simulink model "EffectuatorIntegratedWithDemonstrator"  (R2020a)
settings: Solver=FixedStepDiscrete  StartTime=0.0  StopTime=inf  FixedStep=Ts  RelTol=1e-3
InitFcn:
  | %% Verwende vordefinierte Setpoints (Kreis mit Z-Komponente)
  | 
  | % Config
  | numCircles = 3;
  | scale=6;
  | %Versuch symmetrische Setpunkte zu setzen
  | pointsPerCircle =scale*(4+3*numCircles)+2;
  | 
  | r = 50;
  | m_x = r;
  | m_y = r;
  | 
  | % //
  | s = linspace(0,2*pi,pointsPerCircle);
  | 
  | setPoints_x = [];
  | setPoints_y = [];
  | 
  | for ii=1:numCircles
  | 
  | setPoints_x = [setPoints_x (-cos(s(1:floor(pointsPerCircle / 2))).*r + m_x + 2*r*(ii-1))]; %#ok<AGROW>
  | setPoints_y = [setPoints_y (sin(s).*r+m_y)]; %#ok<AGROW>pointsPerCircle / 2
  | 
  | end
  | 
  | setPoints_x = [setPoints_x flip(setPoints_x(1:end))];
  | 
  | % Loeschen doppelter y-Werte (Kreisuebergang)
  | setPoints_x(pointsPerCircle .* [1:numCircles]) = [];
  | setPoints_y(pointsPerCircle .* [1:numCircles]) = [];
  | 
  | % setPoints_x= [linspace(0,setPoints_x(19),19) setPoints_x(20:end)];
  | % setPoints_y= [linspace(0,setPoints_y(19),19) setPoints_y(20:end)];
  | 
  | % Array Elemente verschieben
  | % setPoints_x = circshift(setPoints_x,-pointsPerCircle/4,2);
  | % setPoints_y = circshift(setPoints_y,-pointsPerCircle/4,2);
  | 
  | z = zeros(1,size(setPoints_x,2));
  | z_x = -5:5;
  | z_y = -z_x.^2 + 25;
  | z_idx = 90;
  | z_idx2 = 210;
  | z(z_idx:z_idx+length(z_x)-1) = z_y;
  | z(z_idx2:z_idx2+length(z_x)-1) = z_y;
  | % z = [z_y z];
  | setPoints_z = z;
  | 
  | % setPoints_x = [zeros(1,length(z_y)) setPoints_x];
  | % setPoints_y = [setPoints_y(1,1)*ones(1,length(z_y)) setPoints_y];
  | 
  | % Umrechnung der Einheiten für Demonstrator
  | % setPoints_x = setPoints_x ./ 1000;
  | % setPoints_y = setPoints_y ./ 1000;
  | % setPoints_z = setPoints_z ./ 1000;
  | 
  | 
  | %{
  | plot(setPoints_x,setPoints_y);
  | fig = figure;
  | ... (+13 lines)
StartFcn:
  | close all;
model workspace (MAT data in the model file):
  MvmtPerfEval_collectVal : Simulink.Parameter (value not decoded)
  MvmtPerfEval_sendOwnVal : Simulink.Parameter (value not decoded)
  PerfEval_numTicks_enable : Simulink.Parameter (value not decoded)
  Segmentregler_I_Gain : Simulink.Parameter (value not decoded)
  Segmentregler_P_Gain : Simulink.Parameter (value not decoded)
  Segmentregler_minVel_enable : Simulink.Parameter (value not decoded)
  Segmentregler_numTicks_enable : Simulink.Parameter (value not decoded)
  Ts : Simulink.Parameter (value not decoded)
  maxPos_x : Simulink.Parameter (value not decoded)
  maxPos_y : Simulink.Parameter (value not decoded)
  maxPos_z : Simulink.Parameter (value not decoded)
  maxVectorLengths : Simulink.Parameter (value not decoded)
  minAllowedVelSaturation : Simulink.Parameter (value not decoded)
  numAxes : Simulink.Parameter (value not decoded)
symbols that are objects in the model workspace (value not decoded): maxPos_x, maxPos_y, maxPos_z, minAllowedVelSaturation, MvmtPerfEval_collectVal, MvmtPerfEval_sendOwnVal, numAxes, PerfEval_numTicks_enable, Segmentregler_I_Gain, Segmentregler_minVel_enable, Segmentregler_numTicks_enable, Segmentregler_P_Gain, Ts
undefined symbols (not defined in the file or in its folder): DiscIntNeverNeededParam, VelOverride
libraries: simulink x20, vrlib x5, sldrtlib x2, xpcrtudplib x2, dspnetwork x2, ptplib x1, etargetslib x1, xpcutilitieslib x1
(part 3 of 5)

== system EffectuatorIntegratedWithDemonstrator/Joystick Ctrl ==
  note: x-Achse
  note: y-Achse
  note: z-Achse
  Custom Gauge : CustomGaugeBlock  LabelPosition=Hide  NeedleImage=data:image/svg+xml;base64,PD94bWwgdmVyc2lvbj0iMS4wIiBlbmNvZGluZz0idXRmLTgiPz4KPCEtLSBHZW5lcmF0b3I6IEFkb2JlIElsbHVzdHJhdG9yIDE5LjIuMSwgU1ZHIEV4cG9ydCBQbHVnLUluIC4gU1ZHIFZlcnNpb246IDYuMDAgQnVpbGQgMCkgIC0tPgo8c3ZnIHZlcnNpb249IjEuMSIgeG1sbnM9Imh0dHA6Ly93d3cudzMub3JnLzIwMDAvc3ZnIiB4bWxuczp4bGluaz0iaHR0cDovL3d3dy53My5vcmcvMTk5OS94bGluayIgeD0iMHB4IiB5PSIwcHgiCgkgdmlld0JveD0iMCAwIDIwMCA1MCIgc3R5bGU9ImVuYWJsZS1iYWNrZ3JvdW5kOm5ldyAw ...(+9940 chars)  NeedleXPos=0.37269714818065863  NeedleYPos=0.4799889804603517  NeedleHeight=0.12331842798957203  NeedleWidth=0.20315800404452888  NeedleInitialRotation=-59.94322499147643  GaugeMax=1  GaugeArcDefined=true  GaugeArcRadius=0.14440076769366753  GaugeArcStrokeWidth=0.042228358658436646  GaugeArcRotation=240.5385250290321  GaugeArcRatio=0.8333333333333  GaugeArcTransparency=0  ValueArcTransparency=0  ValueArcColor=#1759b0  GaugeTickColor=#000000  ScaleColorsJSON=[]  IsLinearGauge=false  GaugeTrackLeft=0.35  GaugeTrackTop=0.35  GaugeTrackHeight=0.1  GaugeTrackWidth=0.3  GaugeTrackRotation=0
  Custom Gauge1 : CustomGaugeBlock  LabelPosition=Hide  GaugeMax=1  GaugeArcDefined=true  GaugeArcRadius=0.1358563990074277  GaugeArcStrokeWidth=0.03972965542329953  GaugeArcRotation=240.5385250290321  GaugeArcRatio=0.8333333333333  GaugeArcTransparency=0  ValueArcColor=#1759b0  GaugeTickColor=#000000  ScaleColorsJSON=[]  IsLinearGauge=false  GaugeTrackLeft=0.35  GaugeTrackTop=0.35  GaugeTrackHeight=0.1  GaugeTrackWidth=0.3  GaugeTrackRotation=0
  Custom Gauge2 : CustomGaugeBlock  LabelPosition=Hide  GaugeMax=1  GaugeArcDefined=true  GaugeArcRadius=0.1358563990074277  GaugeArcStrokeWidth=0.03972965542329953  GaugeArcRotation=240.5385250290321  GaugeArcRatio=0.8333333333333  GaugeArcTransparency=0  ValueArcColor=#1759b0  GaugeTickColor=#000000  ScaleColorsJSON=[]  IsLinearGauge=false  GaugeTrackLeft=0.35  GaugeTrackTop=0.35  GaugeTrackHeight=0.1  GaugeTrackWidth=0.3  GaugeTrackRotation=0
  Custom Gauge3 : CustomGaugeBlock  LabelPosition=Hide  GaugeMax=1  GaugeArcDefined=true  GaugeArcRadius=0.1358563990074277  GaugeArcStrokeWidth=0.03972965542329953  GaugeArcRotation=240.5385250290321  GaugeArcRatio=0.8333333333333  GaugeArcTransparency=0  ValueArcColor=#1759b0  GaugeTickColor=#000000  ScaleColorsJSON=[]  IsLinearGauge=false  GaugeTrackLeft=0.35  GaugeTrackTop=0.35  GaugeTrackHeight=0.1  GaugeTrackWidth=0.3  GaugeTrackRotation=0
  Custom Gauge4 : CustomGaugeBlock  LabelPosition=Hide  NeedleImage=data:image/svg+xml;base64,PD94bWwgdmVyc2lvbj0iMS4wIiBlbmNvZGluZz0idXRmLTgiPz4KPCEtLSBHZW5lcmF0b3I6IEFkb2JlIElsbHVzdHJhdG9yIDE5LjIuMSwgU1ZHIEV4cG9ydCBQbHVnLUluIC4gU1ZHIFZlcnNpb246IDYuMDAgQnVpbGQgMCkgIC0tPgo8c3ZnIHZlcnNpb249IjEuMSIgeG1sbnM9Imh0dHA6Ly93d3cudzMub3JnLzIwMDAvc3ZnIiB4bWxuczp4bGluaz0iaHR0cDovL3d3dy53My5vcmcvMTk5OS94bGluayIgeD0iMHB4IiB5PSIwcHgiCgkgdmlld0JveD0iMCAwIDIwMCA1MCIgc3R5bGU9ImVuYWJsZS1iYWNrZ3JvdW5kOm5ldyAw ...(+9940 chars)  NeedleXPos=0.39476499003029264  NeedleYPos=0.4834578737973021  NeedleHeight=0.10194128264579512  NeedleWidth=0.16794073561990416  NeedleInitialRotation=-59.94322499147643  GaugeMax=1  GaugeArcDefined=true  GaugeArcRadius=0.11936901656721359  GaugeArcStrokeWidth=0.034908108348832664  GaugeArcRotation=240.5385250290321  GaugeArcRatio=0.8333333333333  GaugeArcTransparency=0  ValueArcTransparency=0  ValueArcColor=#1759b0  GaugeTickColor=#000000  ScaleColorsJSON=[]  IsLinearGauge=false  GaugeTrackLeft=0.35  GaugeTrackTop=0.35  GaugeTrackHeight=0.1  GaugeTrackWidth=0.3  GaugeTrackRotation=0
  Custom Gauge5 : CustomGaugeBlock  LabelPosition=Hide  NeedleImage=data:image/svg+xml;base64,PD94bWwgdmVyc2lvbj0iMS4wIiBlbmNvZGluZz0idXRmLTgiPz4KPCEtLSBHZW5lcmF0b3I6IEFkb2JlIElsbHVzdHJhdG9yIDE5LjIuMSwgU1ZHIEV4cG9ydCBQbHVnLUluIC4gU1ZHIFZlcnNpb246IDYuMDAgQnVpbGQgMCkgIC0tPgo8c3ZnIHZlcnNpb249IjEuMSIgeG1sbnM9Imh0dHA6Ly93d3cudzMub3JnLzIwMDAvc3ZnIiB4bWxuczp4bGluaz0iaHR0cDovL3d3dy53My5vcmcvMTk5OS94bGluayIgeD0iMHB4IiB5PSIwcHgiCgkgdmlld0JveD0iMCAwIDIwMCA1MCIgc3R5bGU9ImVuYWJsZS1iYWNrZ3JvdW5kOm5ldyAw ...(+9940 chars)  NeedleXPos=0.38506686522026445  NeedleYPos=0.48193340390288963  NeedleHeight=0.11133586799032906  NeedleWidth=0.18341762126089606  NeedleInitialRotation=-59.94322499147643  GaugeMax=1  GaugeArcDefined=true  GaugeArcRadius=0.1303696866051831  GaugeArcStrokeWidth=0.03812512891780894  GaugeArcRotation=240.5385250290321  GaugeArcRatio=0.8333333333333  GaugeArcTransparency=0  ValueArcTransparency=0  ValueArcColor=#1759b0  GaugeTickColor=#000000  ScaleColorsJSON=[]  IsLinearGauge=false  GaugeTrackLeft=0.35  GaugeTrackTop=0.35  GaugeTrackHeight=0.1  GaugeTrackWidth=0.3  GaugeTrackRotation=0
  Fetch_Global_Data : Subsystem
  Joystick : Subsystem  Commented=on
  Slider : SliderBlock  LabelPosition=Hide  ScaleMax=1  TickInterval=0.2
  Slider1 : SliderBlock  LabelPosition=Hide  ScaleMax=1  TickInterval=0.2
  Slider2 : SliderBlock  LabelPosition=Hide  ScaleMax=1  TickInterval=0.2
  Sliders : Subsystem

== system EffectuatorIntegratedWithDemonstrator/udp_communication ==
  setPoints : Inport
  In1 : Inport  Port=2
  messageToEffectuator : Inport  Port=3
  messageToEffectuator1 : Inport  Port=4
  Communication stack : Subsystem
  Constant : Constant  Commented=on  Value=[230,190,110,70,110,190,linspace(230,725,10),230;75,5,5,75,145,145,75,linspace(75,75,10);4,4,0,0,0,4,4,3,2,1,0,0,1,2,3,4,4];  OutDataTypeStr=int32
  Constant1 : Constant  Commented=on  Value=[0,0,0,0,0,0,0,8,11,11,11,11,0,0,0,0;7,7,7,7,3,3,3,3,7,7,7,7,3,3,3,3;7,7,7,7,3,3,3,3,12,12,7,7,3,3,3,3;8,88,8,7,3,3,3,3,7,7,7,7,3,3,3,3;7,7,7,7,3,3,3,3,7,7,7,7,3,3,6,6];  OutDataTypeStr=int32
  Constant2 : Constant  Commented=on  Value=[230,190,110,70,110,190,linspace(230,725,10),230;75,5,5,75,145,145,75,linspace(75,75,10);4,4,0,0,0,4,4,3,2,1,0,0,1,2,3,4,4];  OutDataTypeStr=int32
  Constant3 : Constant  Commented=on  Value=[0,0,0,0,0,0,0,8,11,11,11,11,0,0,0,0;7,7,7,7,3,3,3,3,7,7,7,7,3,3,3,3;7,7,7,7,3,3,3,3,12,12,7,7,3,3,3,3;8,88,8,7,3,3,3,3,7,7,7,7,3,3,3,3;7,7,7,7,3,3,3,3,7,7,7,7,3,3,6,6];  OutDataTypeStr=int32
  Delay{1..4} (4 alike) : Delay  DelayLength=1
  Display : Display  Commented=on
  Display3 : Display  Commented=on
  MATLAB Function : MATLAB Function  Commented=on  TreatAsAtomicUnit=on
  UDP Send/Receive : Subsystem  TreatAsAtomicUnit=on
  Out1 : Outport
  Out2 : Outport  Port=2
  Out3 : Outport  Port=3
  EffSegmentData : Outport  Port=4
  EffSegmentData1 : Outport  Port=5
  wires:
  MATLAB Function/3(massageReceived) -> Display3/1
  Constant/1 -> MATLAB Function/1(setPoints)
  Constant1/1 -> MATLAB Function/2(kooVec)
  MATLAB Function/2(massageSent) -> Display/1
  UDP Send/Receive/2(messageToEffectuator3) -> Delay1/1
  UDP Send/Receive/3(messageToEffectuator4) -> Delay4/1
  setPoints/1 -> Communication stack/1(setPoints)
  In1/1 -> Communication stack/2(In1)
  Communication stack/1(Out1) -> Out1/1
  Communication stack/2(Out2) -> Out2/1
  Communication stack/3(output) -> Delay3/1
  Communication stack/4(Out3) -> Out3/1
  Communication stack/5(EffSegmentData) -> EffSegmentData/1
  messageToEffectuator/1 -> Communication stack/3(messageToEffectuator)
  messageToEffectuator1/1 -> Communication stack/4(messageToEffectuator1)
  Communication stack/6(output1) -> UDP Send/Receive/Trigger
  Delay4/1 -> Communication stack/7(messageToEffectuator4)
  Delay1/1 -> Communication stack/6(messageToEffectuator3)
  UDP Send/Receive/1(messageToEffectuator2) -> Delay2/1
  Delay3/1 -> UDP Send/Receive/1(In1)
  Delay2/1 -> Communication stack/5(messageToEffectuator2), EffSegmentData1/1

== system EffectuatorIntegratedWithDemonstrator/Achse X/Sat_maxGeschw ==
  Threshold : Inport
  In : Inport  Port=2
  Threshold1 : Inport  Port=3
  Abs : Abs
  Constant : Constant  Value=0
  Multiply : Gain  Gain=-1
  Sign : Signum
  Sum3 : Sum  Inputs=-+
  Switch : Switch  Criteria=u2 > Threshold
  Switch1 : Switch
  Switch2 : Switch  Criteria=u2 > Threshold
  Out : Outport  VectorParamsAs1DForOutWhenUnconnected=off
  wires:
  Multiply/1 -> Switch1/3
  Switch/1 -> Switch1/1, Multiply/1
  Sign/1 -> Switch1/2
  In/1 -> Abs/1, Sign/1
  Abs/1 -> Switch/3, Sum3/2
  Threshold/1 -> Sum3/1, Switch/1
  Sum3/1 -> Switch/2
  Threshold1/1 -> Switch2/2
  Switch1/1 -> Switch2/1
  Constant/1 -> Switch2/3
  Switch2/1 -> Out/1

== system EffectuatorIntegratedWithDemonstrator/Achse X/Sat_sollGeschw ==
  Threshold : Inport
  In : Inport  Port=2
  Abs : Abs
  Constant : Constant  Value=minAllowedVelSaturation
  Display : Display
  Display1 : Display
  Display2 : Display
  Max : MinMax  Function=max  Inputs=2
  Multiply : Gain  Gain=-1
  Sign : Signum
  Sum3 : Sum  Inputs=-+
  Switch : Switch  Criteria=u2 > Threshold
  Switch1 : Switch
  Out : Outport  VectorParamsAs1DForOutWhenUnconnected=off
  wires:
  Sum3/1 -> Switch/2
  Max/1 -> Display1/1, Switch/1, Sum3/1
  Abs/1 -> Sum3/2, Switch/3
  In/1 -> Sign/1, Abs/1
  Sign/1 -> Display2/1, Switch1/2
  Switch/1 -> Multiply/1, Switch1/1
  Multiply/1 -> Switch1/3
  Switch1/1 -> Out/1
  Threshold/1 -> Max/1
  Constant/1 -> Display/1, Max/2

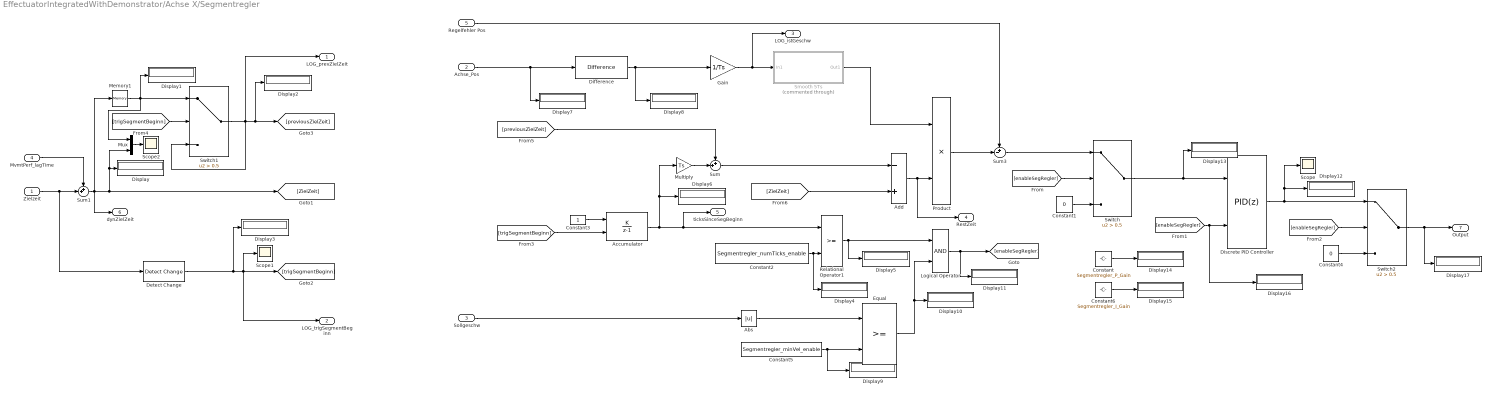
== system EffectuatorIntegratedWithDemonstrator/Achse X/Segmentregler ==
  Zielzeit : Inport
  Achse_Pos : Inport  Port=2
  Sollgeschw : Inport  Port=3
  MvmtPerf_lagTime : Inport  Port=4
  Regelfehler Pos : Inport  Port=5
  Abs : Abs
  Accumulator : DiscreteIntegrator  IntegratorMethod=Accumulation: Forward Euler  gainval=1  ExternalReset=rising  SampleTime=-1  ICPrevOutput=DiscIntNeverNeededParam  ICPrevScaledInput=DiscIntNeverNeededParam
  Add : Sum  Inputs=-+
  Constant : Constant  Value=Segmentregler_P_Gain
  Constant1 : Constant  Value=0
  Constant2 : Constant  Value=Segmentregler_numTicks_enable
  Constant3 : Constant
  Constant4 : Constant  Value=0
  Constant5 : Constant  Value=Segmentregler_minVel_enable
  Constant6 : Constant  Value=Segmentregler_I_Gain
  Detect Change : simulink/Logic and Bit Operations/Detect Change  vinit=0  OutDataTypeStr=boolean
  Difference : simulink/Discrete/Difference  ICPrevInput=0.0  OutMin=[]  OutMax=[]  OutDataType=fixdt(1, 16)  OutScaling=2^-10  DoSatur=off
  Discrete PID Controller : simulink/Continuous/PID Controller  Controller=PID  Form=Parallel  TimeDomain=Discrete-time  UseExternalTs=off  SampleTime=-1  IntegratorMethod=Forward Euler  FilterMethod=Forward Euler  ControllerParametersSource=internal  P=Segmentregler_P_Gain  I=Segmentregler_I_Gain  D=0  UseFilter=on  N=100  TunerSelectOption=Transfer Function Based (PID Tuner App)  InitialConditionSource=internal  InitialConditionForIntegrator=0  InitialConditionForFilter=0  DifferentiatorICPrevScaledInput=0  ExternalReset=falling  TrackingMode=off  Kt=1  LimitOutput=off  UpperSaturationLimit=inf  LowerSaturationLimit=-inf  LinearizeAsGain=off  AntiWindupMode=none  Kb=1  POutMin=[]  POutMax=[]  IOutMin=[]  IOutMax=[]  DOutMin=[]  DOutMax=[]  NOutMin=[]  NOutMax=[]  SumOutMin=[]  SumOutMax=[]  SaturationOutMin=[]  SaturationOutMax=[]  PParamMin=[]  PParamMax=[]  IParamMin=[]  IParamMax=[]  DParamMin=[]  DParamMax=[]  NParamMin=[]  NParamMax=[]  KbParamMin=[]  KbParamMax=[]  KtParamMin=[]  KtParamMax=[]  KbOutMin=[]  KbOutMax=[]  KtOutMin=[]  KtOutMax=[]  IntegratorOutMin=[]  IntegratorOutMax=[]  FilterOutMin=[]  FilterOutMax=[]  SumI1OutMin=[]  SumI1OutMax=[]  SumI2OutMin=[]  SumI2OutMax=[]  SumI3OutMin=[]  SumI3OutMax=[]  SumI4OutMin=[]  SumI4OutMax=[]  SumDOutMin=[]  SumDOutMax=[]  DifferentiatorOutMin=[]  DifferentiatorOutMax=[]  FilterDiffOutCoefMin=[]  FilterDiffOutCoefMax=[]  ReciprocalOutMin=[]  ReciprocalOutMax=[]  SumDenOutMin=[]  SumDenOutMax=[]  SumNumOutMin=[]  SumNumOutMax=[]  DivideOutMin=[]  DivideOutMax=[]  UdiffTsProdOutMin=[]  UdiffTsProdOutMax=[]  NTsProdOutMin=[]  NTsProdOutMax=[]  UintegralTsProdOutMin=[]  UintegralTsProdOutMax=[]  UngainTsProdOutMin=[]  UngainTsProdOutMax=[]  IntegratorContinuousStateAttributes=''  IntegratorStateMustResolveToSignalObject=off  IntegratorRTWStateStorageClass=Auto  FilterContinuousStateAttributes=''  FilterStateMustResolveToSignalObject=off  FilterRTWStateStorageClass=Auto  ParallelPVariant=InternalParameters  IdealPVariant=Disabled  IVariant=InternalParameters  DVariant=InternalParameters  IntegratorVariant=Discrete  SatVariant=Disabled  AWVariant=Passthrough  PCopyVariant=Disabled  TRVariant=Disabled  FdbkBlocksVariant=Forward  IdealPFdbkVariant=Disabled  SatFdbkVariant=Disabled  DerivativeFilterVariant=ForwardEulerFilter  NVariant=InternalParameters  NCopyVariant=Disabled  FilterICVariant=InternalICsFilter  IntegratorICVariant=InternalICs  ExternalResetVariant=ExternalReset  TRSumVariant=Passthrough  SumFdbkVariant=Disabled  SumVariant=Sum_PID  TsampFilterVariant=InternalTs  TsampNgainVariant=Passthrough  TsampIntegralVariant=Passthrough
  Display{,1..17} (18 alike) : Display
  Equal : RelationalOperator  OutDataTypeStr=boolean  RndMeth=Simplest
  Gain : Gain  Gain=1/Ts
  Logical Operator : Logic  AllPortsSameDT=off  OutDataTypeStr=boolean
  Memory1 : Memory
  Multiply : Gain  Gain=Ts
  Mux : Mux  Inputs=2
  Product : Product
  Relational Operator1 : RelationalOperator  OutDataTypeStr=boolean  RndMeth=Simplest
  Scope : Scope
  Scope1 : Scope
  Scope2 : Scope
  Smooth 5Ts : Subsystem  Commented=through
  Sum : Sum  Inputs=++|
  Sum1 : Sum  Inputs=++|
  Sum3 : Sum  Inputs=+-|
  Switch : Switch  Criteria=u2 > Threshold  Threshold=0.5
  Switch1 : Switch  Criteria=u2 > Threshold  Threshold=0.5
  Switch2 : Switch  Criteria=u2 > Threshold  Threshold=0.5
  LOG_prevZielZeit : Outport  VectorParamsAs1DForOutWhenUnconnected=off
  LOG_trigSegmentBeginn : Outport  Port=2  VectorParamsAs1DForOutWhenUnconnected=off
  LOG_istGeschw : Outport  Port=3  VectorParamsAs1DForOutWhenUnconnected=off
  RestZeit : Outport  Port=4  VectorParamsAs1DForOutWhenUnconnected=off
  ticksSinceSegBeginn : Outport  Port=5  VectorParamsAs1DForOutWhenUnconnected=off
  dynZielZeit : Outport  Port=6  VectorParamsAs1DForOutWhenUnconnected=off
  Output : Outport  Port=7  VectorParamsAs1DForOutWhenUnconnected=off
  wires:
  Constant3/1 -> Accumulator/1
  Difference/1 -> Display8/1, Gain/1
  Sum3/1 -> Switch/1
  Switch/1 -> Display13/1, Discrete PID Controller/1
  Sum/1 -> Add/1
  Relational Operator1/1 -> Display5/1, Logical Operator/1
  Add/1 -> RestZeit/1, Product/2
  Constant2/1 -> Display4/1, Relational Operator1/2
  Achse_Pos/1 -> Display7/1, Difference/1
  Discrete PID Controller/1 -> Display12/1, Scope/1, Switch2/1
  Constant1/1 -> Switch/3
  Constant4/1 -> Switch2/3
  Product/1 -> Sum3/2
  Regelfehler Pos/1 -> Sum3/1
  Switch2/1 -> Display17/1, Output/1
  Logical Operator/1 -> Display11/1, [enableSegRegler]
  [enableSegRegler] -> Switch/2
  [enableSegRegler] -> Switch2/2
  Sollgeschw/1 -> Abs/1
  Constant5/1 -> Display9/1, Equal/2
  Equal/1 -> Display10/1, Logical Operator/2
  Sum1/1 -> Memory1/1, Mux/2, Display/1, [ZielZeit], dynZielZeit/1
  Gain/1 -> LOG_istGeschw/1, Smooth 5Ts/1(In1)
  Detect Change/1 -> Display3/1, Scope1/1, LOG_trigSegmentBeginn/1, [trigSegmentBeginn]
  [trigSegmentBeginn] -> Switch1/2
  Switch1/1 -> Display2/1, [previousZielZeit], Switch1/3, LOG_prevZielZeit/1
  [previousZielZeit] -> Sum/1
  Smooth 5Ts/1(Out1) -> Product/1
  Multiply/1 -> Sum/2
  [ZielZeit] -> Add/2
  Abs/1 -> Equal/1
  Zielzeit/1 -> Detect Change/1, Sum1/2
  MvmtPerf_lagTime/1 -> Sum1/1
  Accumulator/1 -> Display6/1, Multiply/1, ticksSinceSegBeginn/1, Relational Operator1/1
  [trigSegmentBeginn] -> Accumulator/2
  Constant/1 -> Display14/1
  Constant6/1 -> Display15/1
  [enableSegRegler] -> Display16/1, Discrete PID Controller/2
  Mux/1 -> Scope2/1
  Memory1/1 -> Mux/1, Display1/1, Switch1/1
